simulink model "Exhaust_Aftertreatment_System_Model"  (R2016b)
settings: Solver=FixedStepDiscrete  StartTime=0.0  StopTime=inf  FixedStep=ExhATSysMdl.tiSimnTiStep_C.Value  RelTol=1e-3  EnableMultiTasking=on
settings Model: SimulationMode=accelerator  Creator=mmichlin  LastModifiedBy=mmichlin
settings DebuggingCC: SignalInfNanChecking=warning  ReadBeforeWriteMsg=DisableAll  WriteAfterWriteMsg=EnableAllAsWarning  WriteAfterReadMsg=DisableAll  InheritedTsInSrcMsg=none  MultiTaskRateTransMsg=warning  Int32ToFloatConvMsg=none  ParameterOverflowMsg=warning  ParameterPrecisionLossMsg=none  FcnCallInpInsideContextMsg=warning  UnconnectedInputMsg=error  UnconnectedOutputMsg=error  UniqueDataStoreMsg=error  StateNameClashWarn=warning  SFUnexpectedBacktrackingDiag=warning  SFNoUnconditionalDefaultTransitionDiag=warning  SFExecutionAtInitializationDiag=none  UnitsInconsistencyMsg=none
settings ModelReferenceCC: PropagateSignalLabelsOutOfModel=off
settings GRTTargetCC: TargetLangStandard=C89/C90 (ANSI)

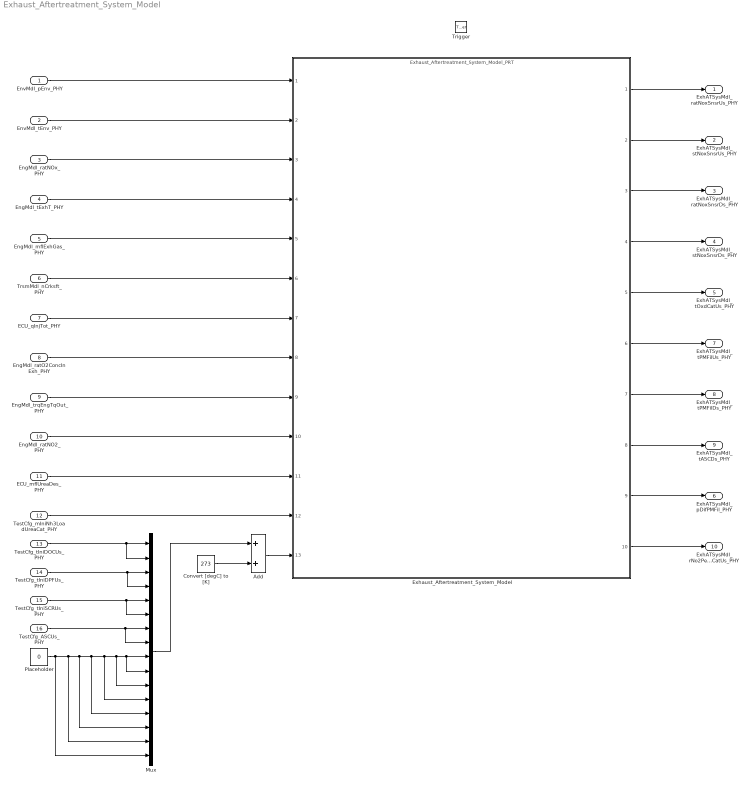
== system Exhaust_Aftertreatment_System_Model ==
  EnvMdl_pEnv_PHY : Inport
  EnvMdl_tEnv_PHY : Inport  Port=2
  EngMdl_ratNOx_PHY : Inport  Port=3
  EngMdl_tExhT_PHY : Inport  Port=4
  EngMdl_mflExhGas_PHY : Inport  Port=5
  TrsmMdl_nCrksft_PHY : Inport  Port=6
  ECU_qInjTot_PHY : Inport  Port=7
  EngMdl_ratO2ConcInExh_PHY : Inport  Port=8
  EngMdl_trqEngTqOut_PHY : Inport  Port=9
  EngMdl_ratNO2_PHY : Inport  Port=10
  ECU_mflUreaDes_PHY : Inport  Port=11
  TestCfg_mIniNh3LoadUreaCat_PHY : Inport  Port=12
  TestCfg_tIniDOCUs_PHY : Inport  Port=13
  TestCfg_tIniDPFUs_PHY : Inport  Port=14
  TestCfg_tIniSCRUs_PHY : Inport  Port=15
  TestCfg_ASCUs_PHY : Inport  Port=16
  Trigger : TriggerPort  TriggerType=function-call  VariantControl=Variant  PortDimensions=1
  Add : Sum
  Convert [degC] to [K] : Constant  Value=273
  Exhaust_Aftertreatment_System_Model : ModelReference  ModelNameDialog=Exhaust_Aftertreatment_System_Model_PRT.slxp  ModelReferenceVersion=1.62  CopyOfModelProtected=on
  Mux : Mux  Inputs=16
  Placeholder : Constant  Value=0
  ExhATSysMdl_ratNoxSnsrUs_PHY : Outport
  ExhATSysMdl_stNoxSnsrUs_PHY : Outport  Port=2
  ExhATSysMdl_ratNoxSnsrDs_PHY : Outport  Port=3
  ExhATSysMdl_stNoxSnsrDs_PHY : Outport  Port=4
  ExhATSysMdl_tOxdCatUs_PHY : Outport  Port=5
  ExhATSysMdl_pDifPMFil_PHY : Outport  Port=6
  ExhATSysMdl_tPMFilUs_PHY : Outport  Port=7
  ExhATSysMdl_tPMFilDs_PHY : Outport  Port=8
  ExhATSysMdl_tASCDs_PHY : Outport  Port=9
  ExhATSysMdl_rNo2PerNoxUreaCatUs_PHY : Outport  Port=10
  wires:
  Exhaust_Aftertreatment_System_Model/5 -> ExhATSysMdl_tOxdCatUs_PHY/1
  Exhaust_Aftertreatment_System_Model/9 -> ExhATSysMdl_pDifPMFil_PHY/1
  Exhaust_Aftertreatment_System_Model/6 -> ExhATSysMdl_tPMFilUs_PHY/1
  Exhaust_Aftertreatment_System_Model/7 -> ExhATSysMdl_tPMFilDs_PHY/1
  Exhaust_Aftertreatment_System_Model/8 -> ExhATSysMdl_tASCDs_PHY/1
  ECU_qInjTot_PHY/1 -> Exhaust_Aftertreatment_System_Model/7
  TrsmMdl_nCrksft_PHY/1 -> Exhaust_Aftertreatment_System_Model/6
  EngMdl_tExhT_PHY/1 -> Exhaust_Aftertreatment_System_Model/4
  EngMdl_ratNOx_PHY/1 -> Exhaust_Aftertreatment_System_Model/3
  EnvMdl_tEnv_PHY/1 -> Exhaust_Aftertreatment_System_Model/2
  EngMdl_mflExhGas_PHY/1 -> Exhaust_Aftertreatment_System_Model/5
  EnvMdl_pEnv_PHY/1 -> Exhaust_Aftertreatment_System_Model/1
  EngMdl_ratO2ConcInExh_PHY/1 -> Exhaust_Aftertreatment_System_Model/8
  EngMdl_trqEngTqOut_PHY/1 -> Exhaust_Aftertreatment_System_Model/9
  EngMdl_ratNO2_PHY/1 -> Exhaust_Aftertreatment_System_Model/10
  ECU_mflUreaDes_PHY/1 -> Exhaust_Aftertreatment_System_Model/11
  TestCfg_mIniNh3LoadUreaCat_PHY/1 -> Exhaust_Aftertreatment_System_Model/12
  Exhaust_Aftertreatment_System_Model/1 -> ExhATSysMdl_ratNoxSnsrUs_PHY/1
  Exhaust_Aftertreatment_System_Model/2 -> ExhATSysMdl_stNoxSnsrUs_PHY/1
  Exhaust_Aftertreatment_System_Model/4 -> ExhATSysMdl_stNoxSnsrDs_PHY/1
  Exhaust_Aftertreatment_System_Model/3 -> ExhATSysMdl_ratNoxSnsrDs_PHY/1
  Exhaust_Aftertreatment_System_Model/10 -> ExhATSysMdl_rNo2PerNoxUreaCatUs_PHY/1
  TestCfg_tIniDOCUs_PHY/1 -> Mux/2, Mux/1
  TestCfg_tIniDPFUs_PHY/1 -> Mux/4, Mux/3
  TestCfg_tIniSCRUs_PHY/1 -> Mux/6, Mux/5
  TestCfg_ASCUs_PHY/1 -> Mux/8, Mux/7
  Mux/1 -> Add/1
  Convert [degC] to [K]/1 -> Add/2
  Add/1 -> Exhaust_Aftertreatment_System_Model/13
  Placeholder/1 -> Mux/16, Mux/15, Mux/14, Mux/13, Mux/12, Mux/11, Mux/10, Mux/9
